simulink model "W3prob3"  (R2020b)
settings: Solver=VariableStepAuto  StartTime=0.0  StopTime=10.0  RelTol=1e-3
settings Model: EnablePacing=on  Creator=deves  LastModifiedBy=deves

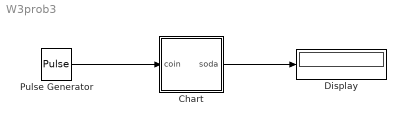
== system W3prob3 ==
  Chart : Stateflow chart  TreatAsAtomicUnit=on
  Display : Display
  Pulse Generator : DiscretePulseGenerator  PulseType=Time based  Period=1  PulseWidth=5
  wires:
  Pulse Generator/1 -> Chart/1(coin)
  Chart/1(soda) -> Display/1

== stateflow chart W3prob3/Chart ==
  state NoNickel
  state Dime_1
  state Nickel_1
  (default) -> NoNickel
  NoNickel -> Dime_1 [order 2] : [coin==2]{soda=0;}
  Nickel_1 -> NoNickel [order 2] : [coin==2]{soda=1;}
  NoNickel -> Nickel_1 [order 1] : [coin==1]{soda=0;}
  Dime_1 -> NoNickel [order 2] : [coin ==1]{soda=1;}
  Nickel_1 -> Dime_1 [order 1] : [coin==1]{soda=0;}
  Dime_1 -> Nickel_1 [order 1] : [coin==2]{soda=1;}
  data: coin input; soda output
